simulink model "SimplePIDTest"  (R2024b)
settings: Solver=ode45  StartTime=0.0  StopTime=20  RelTol=1e-3
settings Model: Creator=mkozl  LastModifiedBy=mkozl

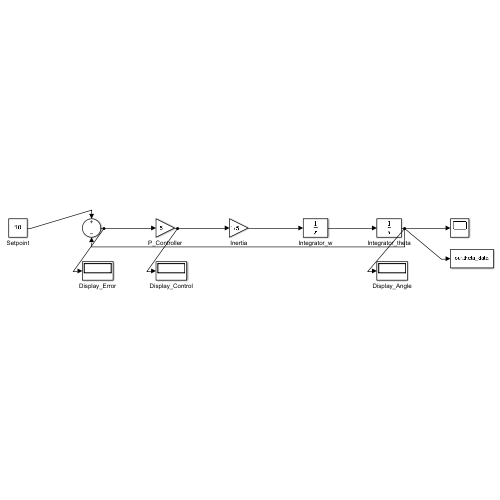
[thumbnail: Simulink's stored preview of the top-level diagram]
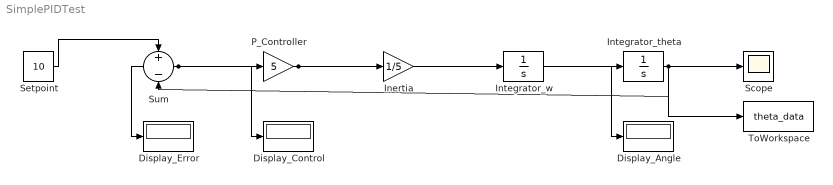
== system SimplePIDTest ==
  Display_Angle : Display
  Display_Control : Display
  Display_Error : Display
  Inertia : Gain  Gain=1/5
  Integrator_theta : Integrator
  Integrator_w : Integrator
  P_Controller : Gain  Gain=5
  Scope : Scope
  Setpoint : Constant  Value=10
  Sum : Sum  Inputs=+-
  ToWorkspace : ToWorkspace  VariableName=theta_data  SaveFormat=Structure With Time  SampleTime=-1
  wires:
  Setpoint/1 -> Sum/1
  Sum/1 -> P_Controller/1, Display_Error/1
  P_Controller/1 -> Inertia/1, Display_Control/1
  Inertia/1 -> Integrator_w/1
  Integrator_w/1 -> Integrator_theta/1
  Integrator_theta/1 -> Scope/1, ToWorkspace/1, Display_Angle/1, Sum/2
